simulink model "Relu_OutFB_4_4_1_HW_C1"  (R2012b)
settings: Solver=FixedStepDiscrete  SolverMode=SingleTasking  StartTime=0.0  StopTime=limSim*buffer  RelTol=1e-3
undefined symbols (not defined in the file): alpha, buffer, delayMulx, delayMuly, delayROMSig, limSim, m, M2, M3, magnitude, mu, n, p, ts
libraries: xbsIndex_r4 x268, dspstat3 x1, roblocks x1
(part 1 of 3)
settings Model: Creator=Marcelo  LastModifiedBy=snata
settings DataIOCC: SignalLoggingSaveFormat=ModelDataLogs
settings DebuggingCC: MultiTaskDSMMsg=warning  MultiTaskCondExecSysMsg=none  FcnCallInpInsideContextMsg=UseLocalSettings  StrictBusMsg=None
settings RTWCC: IncludeERTFirstTime=on
settings CodeAppCC: CustomSymbolStrType=$N$R$M_T  InternalIdentifier=Shortened
settings GRTTargetCC: CombineOutputUpdateFcns=off  GRTInterface=on

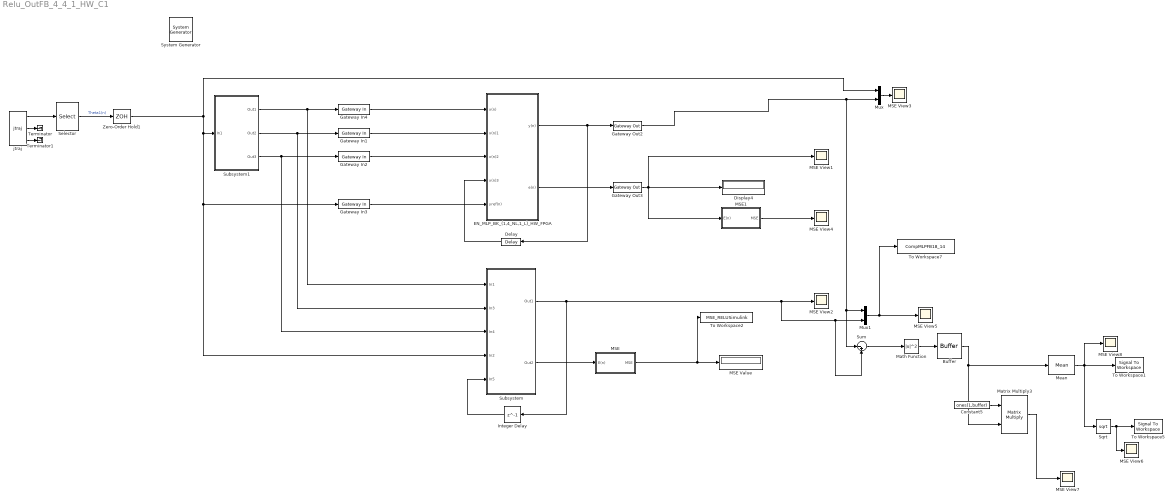
== system Relu_OutFB_4_4_1_HW_C1 ==
  " System Generator" : xbsIndex_r4/ System Generator  Tag=genX  xilinxfamily=virtex6  part=xc6vlx240t  speed=-1  package=ff1156  synthesis_tool=XST  clock_wrapper=Clock Enables  directory=C:/Users/snata/Documents/Netlist_MLP_Relu4_4_1  proj_type=Project Navigator  Synth_file=XST Defaults  Impl_file=ISE Defaults  testbench=off  simulink_period=ts  sysclk_period=10  dcm_input_clock_period=10  incr_netlist=off  trim_vbits=Everywhere in SubSystem  dbl_ovrd=According to Block Masks  core_generation=According to Block Masks  run_coregen=off  deprecated_control=off  eval_field=0  block_type=sysgen
  Buffer : Buffer  N=buffer  TreatMby1Signals=One channel
  Constant5 : Constant  Value=ones(1,buffer)  VectorParams1D=off
  Delay : xbsIndex_r4/Delay  rst=off  infoeditControl=Selection of Reset will increase slice count due to use of real FFs and instead of SRLs  en=off  latency=delayROMSig+delayMulx+delayMuly  dbl_ovrd=off  reg_retiming=off  block_type=delay
  Display4 : Display
  EN_MLP_BK_(1,4_NL,1_L)_HW_FPGA : Subsystem
  Gateway In{1..4} (4 alike) : xbsIndex_r4/Gateway In  gui_display_data_type=Fixed-point  arith_type="Signed  (2's comp)"  n_bits=nb  bin_pt=bp  preci_type=Single  exp_width=8  frac_width=24  quantization="Round  (unbiased: +/- Inf)"  overflow=Saturate  period=ts  dbl_ovrd=off  timing_constraint=None  locs_specified=off  LOCs={}  UseAsADC=off  ADCChannel='1'  inherit_from_input=off  hdl_port=on  block_type=gatewayin
  Gateway Out2 : xbsIndex_r4/Gateway Out  inherit_from_input=off  hdl_port=on  timing_constraint=None  locs_specified=off  LOCs={}  UseAsDAC=off  DACChannel='1'  block_type=gatewayout
      settings: infoedit="Gateway out block.  Converts Xilinx fixed point inputs into ouputs of type Simulink integer, double, or fixed point.<br><br>Hardware notes:  In hardware these blocks become top level output ports or are discarded, depending on how they are configured."
  Gateway Out3 : xbsIndex_r4/Gateway Out  inherit_from_input=off  hdl_port=on  timing_constraint=None  locs_specified=off  LOCs={}  UseAsDAC=off  DACChannel='1'  block_type=gatewayout
      settings: infoedit="Gateway out block.  Converts Xilinx fixed point inputs into ouputs of type Simulink integer, double, or fixed point.<br><br>Hardware notes:  In hardware these blocks become top level output ports or are discarded, depending on how they are configured."
  Integer Delay : Delay  DelayLength=1  InputProcessing=Inherited  SampleTime=ts
  MSE : Subsystem  mask(MSE){N=1, m=1}
      mask prompts: N "training size:"; m "Number of output neurons:"
      mask help:
      | MSE
      |
      | Prof. Marcelo Augusto Costa Fernandes
      | DCA - CT - UFRN
      | mfernandes@dca.ufrn.br
      mask Help:
      | MSE
      | 
      | Prof. Marcelo Augusto Costa Fernandes
      | DCA - CT - UFRN
      | mfernandes@dca.ufrn.br
  MSE Value : Display
  MSE View{1..8} (8 alike) : Scope
      MSE View1 settings: YMin=-70  YMax=70  SaveName=ScopeData2  MaxDataPoints=5000000
      MSE View2 settings: YMin=0.043  YMax=0.066  MaxDataPoints=5000000
      MSE View3 settings: ShowLegends=on  YMin=-70  YMax=70  SaveName=ScopeData7  MaxDataPoints=5000000
      MSE View4 settings: YMin=0.013  YMax=0.025  SaveName=ScopeData3  MaxDataPoints=5000000
      MSE View5 settings: YMin=-70  YMax=70  MaxDataPoints=5000000
      MSE View6 settings: TimeRange=1600  YMin=0.3388218390804599  YMax=0.5988218390804599  SaveName=ScopeData4  MaxDataPoints=5000000
      MSE View7 settings: TimeRange=1600  YMin=0.3388218390804599  YMax=0.5988218390804599  SaveName=ScopeData5  MaxDataPoints=5000000
      MSE View8 settings: TimeRange=1600  YMin=0.3388218390804599  YMax=0.5988218390804599  SaveName=ScopeData6  MaxDataPoints=5000000
  MSE1 : Subsystem  mask(MSE){N=1, m=1}
      mask prompts: N "training size:"; m "Number of output neurons:"
      mask help:
      | MSE
      |
      | Prof. Marcelo Augusto Costa Fernandes
      | DCA - CT - UFRN
      | mfernandes@dca.ufrn.br
      mask Help:
      | MSE
      | 
      | Prof. Marcelo Augusto Costa Fernandes
      | DCA - CT - UFRN
      | mfernandes@dca.ufrn.br
  Math Function : Math  Operator=magnitude^2  SaturateOnIntegerOverflow=on
  Matrix Multiply3 : Product  Multiplication=Matrix(*)
  Mean : dspstat3/Mean  run=off  reset_popup=None  InputProcessing=Columns as channels (frame based)  directionMode=Each column  dimension=1  treatSBRowAsCol=on  roiEnable=off  roiType=Rectangles  roiPortion=Entire ROI  roiOutput=Individual statistics for each ROI  roiFlag=off  outputDataTypeStr=Inherit: Same as accumulator  outputLastDataTypeStr=Inherit: Same as accumulator  outputMin=[]  outputMax=[]  roundingMode=Floor  overflowMode=off
  Mux : Mux  Inputs=2
  Mux1 : Mux  Inputs=2
  Selector : Selector  InputPortWidth=3  IndexOptions=Index vector (dialog)  Indices=[1]  OutputSizes=1
  Sqrt : Sqrt  SaturateOnIntegerOverflow=on
  Subsystem : Subsystem
  Subsystem1 : Subsystem
  Sum : Sum  Inputs=|-+
  Terminator : Terminator
  Terminator1 : Terminator
  To Workspace1 : SignalToWorkspace  VariableName=MSEMLPFB14_10
  To Workspace2 : ToWorkspace  VariableName=MSE_RELUSimulink  SampleTime=-1
  To Workspace5 : SignalToWorkspace  VariableName=RMSEMLPFB14_10
  To Workspace7 : ToWorkspace  VariableName=CompMLPFB18_14  SampleTime=-1
  Zero-Order Hold1 : ZeroOrderHold  SampleTime=ts
  jtraj : roblocks/Trajectory/jtraj  q0=[0 -pi/2 pi]  qf=[pi/2 pi/4 pi/2]  tmax=limSim*buffer  ts=1
  wires:
  jtraj/1 -> Selector/1
  Selector/1 -> Zero-Order Hold1/1  "Theta1(n)"
  jtraj/2 -> Terminator/1
  jtraj/3 -> Terminator1/1
  EN_MLP_BK_(1,4_NL,1_L)_HW_FPGA/2(e(n)) -> Gateway Out3/1
  Gateway In4/1 -> EN_MLP_BK_(1,4_NL,1_L)_HW_FPGA/1(x(n))
  Gateway In3/1 -> EN_MLP_BK_(1,4_NL,1_L)_HW_FPGA/5(yref(n))
  Gateway Out3/1 -> MSE1/1(E(n)), MSE View1/1, Display4/1
  Gateway In1/1 -> EN_MLP_BK_(1,4_NL,1_L)_HW_FPGA/2(x(n)1)
  Gateway In2/1 -> EN_MLP_BK_(1,4_NL,1_L)_HW_FPGA/3(x(n)2)
  MSE1/1(MSE) -> MSE View4/1
  EN_MLP_BK_(1,4_NL,1_L)_HW_FPGA/1(y(n)) -> Delay/1, Gateway Out2/1
  Delay/1 -> EN_MLP_BK_(1,4_NL,1_L)_HW_FPGA/4(x(n)3)
  Mux/1 -> MSE View3/1
  Subsystem1/1(Out1) -> Subsystem/1(In1), Gateway In4/1
  Subsystem1/2(Out2) -> Subsystem/2(In3), Gateway In1/1
  Subsystem1/3(Out3) -> Subsystem/3(In4), Gateway In2/1
  Subsystem/2(Out2) -> MSE/1(E(n))
  Zero-Order Hold1/1 -> Subsystem1/1(In1), Subsystem/4(In2), Gateway In3/1, Mux/1
  Mux1/1 -> MSE View5/1, To Workspace7/1
  MSE/1(MSE) -> To Workspace2/1, MSE Value/1
  Integer Delay/1 -> Subsystem/5(In5)
  Sum/1 -> Math Function/1
  Math Function/1 -> Buffer/1
  Buffer/1 -> Mean/1, Matrix Multiply3/2
  Mean/1 -> MSE View8/1, Sqrt/1, To Workspace1/1
  Matrix Multiply3/1 -> MSE View7/1
  Constant5/1 -> Matrix Multiply3/1
  Sqrt/1 -> MSE View6/1, To Workspace5/1
  Gateway Out2/1 -> Sum/1, Mux1/1, Mux/2
  Subsystem/1(Out1) -> Integer Delay/1, Sum/2, Mux1/2, MSE View2/1

== system Relu_OutFB_4_4_1_HW_C1/EN_MLP_BK_(1,4_NL,1_L)_HW_FPGA ==
  x(n) : Inport
  x(n)1 : Inport  Port=2
  x(n)2 : Inport  Port=3
  x(n)3 : Inport  Port=4
  yref(n) : Inport  Port=5
  MLP_BK_(2,4_NL,1_L)_HW_FPGA : Subsystem
  y(n) : Outport
  e(n) : Outport  Port=2
  wires:
  yref(n)/1 -> MLP_BK_(2,4_NL,1_L)_HW_FPGA/5(y_ref(n))
  x(n)/1 -> MLP_BK_(2,4_NL,1_L)_HW_FPGA/1(x_1(n))  "x(n)"
  MLP_BK_(2,4_NL,1_L)_HW_FPGA/2(e(n)) -> e(n)/1
  x(n)1/1 -> MLP_BK_(2,4_NL,1_L)_HW_FPGA/2(x_2(n))
  x(n)2/1 -> MLP_BK_(2,4_NL,1_L)_HW_FPGA/3(x_3(n))
  MLP_BK_(2,4_NL,1_L)_HW_FPGA/1(y(n)) -> y(n)/1
  x(n)3/1 -> MLP_BK_(2,4_NL,1_L)_HW_FPGA/4(x_4(n))

== system Relu_OutFB_4_4_1_HW_C1/MSE ==
  E(n) : Inport
  Add1 : Sum  Inputs=1
  Constant5 : Constant  Value=ones(1,m)  VectorParams1D=off
  Gain : Gain  Gain=1/N
  Math Function : Math  Operator=magnitude^2  SaturateOnIntegerOverflow=on
  Matrix Multiply3 : Product  Multiplication=Matrix(*)
  MSE : Outport
  wires:
  Add1/1 -> Gain/1
  Constant5/1 -> Matrix Multiply3/1
  Math Function/1 -> Matrix Multiply3/2
  Matrix Multiply3/1 -> Add1/1
  E(n)/1 -> Math Function/1
  Gain/1 -> MSE/1

== system Relu_OutFB_4_4_1_HW_C1/MSE1 ==
  E(n) : Inport
  Add1 : Sum  Inputs=1
  Constant5 : Constant  Value=ones(1,m)  VectorParams1D=off
  Gain : Gain  Gain=1/N
  Math Function : Math  Operator=magnitude^2  SaturateOnIntegerOverflow=on
  Matrix Multiply3 : Product  Multiplication=Matrix(*)
  MSE : Outport
  wires:
  Gain/1 -> MSE/1
  E(n)/1 -> Math Function/1
  Matrix Multiply3/1 -> Add1/1
  Math Function/1 -> Matrix Multiply3/2
  Constant5/1 -> Matrix Multiply3/1
  Add1/1 -> Gain/1

== system Relu_OutFB_4_4_1_HW_C1/Subsystem ==
  In1 : Inport
  In3 : Inport  Port=2
  In4 : Inport  Port=3
  In2 : Inport  Port=4
  In5 : Inport  Port=5
  Add : Sum  Inputs=-+|
  Backpropagation Algorithm : Subsystem  mask(Backpropagation Algorithm){mu=mu, alpha=0, N=1, p=n, H=m, m=p, ts=ts}
      mask prompts: N "training size:"; p "Number of the inputs:"; H "Number of hidden neurons:"; m "Number of output neurons:"; ts "Sample time:"
      mask help:
      | Backpropagation Algorithm
      |
      | Prof. Marcelo A. C. Fernandes
      | DCA - CT - UFRN
      | mfernandes@dca.ufrn.br
      mask Help:
      | Backpropagation Algorithm
      | 
      | Prof. Marcelo A. C. Fernandes
      | DCA - CT - UFRN
      | mfernandes@dca.ufrn.br
  MLP - 2 Layers : Subsystem  mask(Multilayer Perceptron (MLP) - 2 Layers){N=1, valorLimiar=1, p=n, H=m, m=p, ts=ts}
      mask prompts: N "training size:"; valorLimiar "Bias value:"; p "Number of the inputs:"; H "Number of hidden neurons:"; m "Number of output neurons:"; ts "sampleTime"
      mask help:
      | Multilayer Perceptron (MLP) - 2 Layers
      |
      | Prof. Marcelo Augusto Costa Fernandes
      | DCA - CT - UFRN
      | mfernandes@dca.ufrn.br
      mask Help:
      | Multilayer Perceptron (MLP) - 2 Layers
      | 
      | Prof. Marcelo Augusto Costa Fernandes
      | DCA - CT - UFRN
      | mfernandes@dca.ufrn.br
  Matrix Concatenate : Concatenate  NumInputs=4  Mode=Multidimensional array
  Out1 : Outport
  Out2 : Outport  Port=2
  wires:
  MLP - 2 Layers/1(Y(n)) -> Add/1, Out1/1
  In4/1 -> Matrix Concatenate/3
  In3/1 -> Matrix Concatenate/2
  In1/1 -> Matrix Concatenate/1
  In2/1 -> Add/2
  Matrix Concatenate/1 -> MLP - 2 Layers/1(X(n))
  Backpropagation Algorithm/1(Wy(n+1)) -> MLP - 2 Layers/3(Wy(n+1))
  Add/1 -> Out2/1, Backpropagation Algorithm/3(E(n))
  MLP - 2 Layers/2("[bias|Z(n)]") -> Backpropagation Algorithm/2("[bias|Z(n)]")
  MLP - 2 Layers/3("[bias|X(n)]") -> Backpropagation Algorithm/1("[bias|X(n)]")
  In5/1 -> Matrix Concatenate/4
  Backpropagation Algorithm/2(Wx(n+1)) -> MLP - 2 Layers/2(Wx(n+1))

== system Relu_OutFB_4_4_1_HW_C1/Subsystem1 ==
  In1 : Inport
  Delay{1..6} (6 alike) : Delay  DelayLength=1
  Terminator : Terminator
  Out1 : Outport
  Out2 : Outport  Port=2
  Out3 : Outport  Port=3
  wires:
  Delay4/1 -> Delay1/1, Out3/1
  Delay2/1 -> Out2/1, Delay4/1
  Delay3/1 -> Out1/1, Delay2/1
  In1/1 -> Delay3/1
  Delay1/1 -> Delay5/1
  Delay5/1 -> Delay6/1
  Delay6/1 -> Terminator/1

== system Relu_OutFB_4_4_1_HW_C1/EN_MLP_BK_(1,4_NL,1_L)_HW_FPGA/MLP_BK_(2,4_NL,1_L)_HW_FPGA ==
  x_1(n) : Inport
  x_2(n) : Inport  Port=2
  x_3(n) : Inport  Port=3
  x_4(n) : Inport  Port=4
  y_ref(n) : Inport  Port=5
  AddSub : xbsIndex_r4/AddSub  mode=Subtraction  use_carryin=off  use_carryout=off  en=off  latency=0  precision=User Defined  arith_type="Signed  (2's comp)"  n_bits=nb  bin_pt=bp  quantization="Round  (unbiased: +/- Inf)"  overflow=Wrap  dbl_ovrd=off  use_behavioral_HDL=off  hw_selection=Fabric  pipelined=off  block_type=addsub
  BK (2,4_NL,1_L) : Subsystem
  Delay{,1..4} (5 alike) : xbsIndex_r4/Delay  rst=off  infoeditControl=Selection of Reset will increase slice count due to use of real FFs and instead of SRLs  en=off  latency=delayROMSig+delayMulx+delayMuly  dbl_ovrd=off  reg_retiming=off  block_type=delay
  MLP (2,4_NL,1_L) : Subsystem
  y(n) : Outport
  e(n) : Outport  Port=2
  wires:
  Delay/1 -> AddSub/1
  y_ref(n)/1 -> Delay/1
  x_1(n)/1 -> MLP (2,4_NL,1_L)/4(x_1(n))
  BK (2,4_NL,1_L)/1(Wy_10(n)) -> MLP (2,4_NL,1_L)/29(Wy_10(n))
  AddSub/1 -> e(n)/1, BK (2,4_NL,1_L)/11(e(n))
  BK (2,4_NL,1_L)/2(Wy_11(n)) -> MLP (2,4_NL,1_L)/28(Wy_11(n))
  x_2(n)/1 -> MLP (2,4_NL,1_L)/3(x_2(n))
  x_3(n)/1 -> MLP (2,4_NL,1_L)/2(x_3(n))
  x_4(n)/1 -> MLP (2,4_NL,1_L)/1(x_4(n))
  BK (2,4_NL,1_L)/3(Wy_12(n)) -> MLP (2,4_NL,1_L)/27(Wy_12(n))
  BK (2,4_NL,1_L)/4(Wy_13(n)) -> MLP (2,4_NL,1_L)/26(Wy_13(n))
  BK (2,4_NL,1_L)/5(Wy_14(n)) -> MLP (2,4_NL,1_L)/25(Wy_14(n))
  BK (2,4_NL,1_L)/6(Wx_10(n)) -> MLP (2,4_NL,1_L)/24(Wx_10(n))
  BK (2,4_NL,1_L)/7(Wx_11(n)) -> MLP (2,4_NL,1_L)/23(Wx_11(n))
  BK (2,4_NL,1_L)/8(Wx_12(n)) -> MLP (2,4_NL,1_L)/22(Wx_12(n))
  BK (2,4_NL,1_L)/9(Wx_13(n)) -> MLP (2,4_NL,1_L)/21(Wx_13(n))
  BK (2,4_NL,1_L)/10(Wx_14(n)) -> MLP (2,4_NL,1_L)/20(Wx_14(n))
  BK (2,4_NL,1_L)/11(Wx_20(n)) -> MLP (2,4_NL,1_L)/19(Wx_20(n))
  BK (2,4_NL,1_L)/12(Wx_21(n)) -> MLP (2,4_NL,1_L)/18(Wx_21(n))
  BK (2,4_NL,1_L)/13(Wx_22(n)) -> MLP (2,4_NL,1_L)/17(Wx_22(n))
  BK (2,4_NL,1_L)/14(Wx_23(n)) -> MLP (2,4_NL,1_L)/16(Wx_23(n))
  BK (2,4_NL,1_L)/15(Wx_24(n)) -> MLP (2,4_NL,1_L)/15(Wx_24(n))
  BK (2,4_NL,1_L)/16(Wx_30(n)) -> MLP (2,4_NL,1_L)/14(Wx_30(n))
  BK (2,4_NL,1_L)/17(Wx_31(n)) -> MLP (2,4_NL,1_L)/13(Wx_31(n))
  BK (2,4_NL,1_L)/18(Wx_32(n)) -> MLP (2,4_NL,1_L)/12(Wx_32(n)1)
  BK (2,4_NL,1_L)/19(Wx_33(n)) -> MLP (2,4_NL,1_L)/11(Wx_33(n))
  BK (2,4_NL,1_L)/20(Wx_34(n)) -> MLP (2,4_NL,1_L)/10(Wx_34(n))
  BK (2,4_NL,1_L)/21(Wx_40(n)) -> MLP (2,4_NL,1_L)/9(Wx_40(n))
  BK (2,4_NL,1_L)/22(Wx_41(n)) -> MLP (2,4_NL,1_L)/8(Wx_41(n))
  BK (2,4_NL,1_L)/23(Wx_42(n)) -> MLP (2,4_NL,1_L)/7(Wx_42(n))
  BK (2,4_NL,1_L)/24(Wx_43(n)) -> MLP (2,4_NL,1_L)/6(Wx_43(n))
  BK (2,4_NL,1_L)/25(Wx_44(n)) -> MLP (2,4_NL,1_L)/5(Wx_44(n))
  MLP (2,4_NL,1_L)/11(x_4(n)bp) -> Delay1/1
  MLP (2,4_NL,1_L)/10(x_3(n)bp) -> Delay2/1
  MLP (2,4_NL,1_L)/9(x_2(n)bp) -> Delay3/1
  MLP (2,4_NL,1_L)/8(x_1(n)bp) -> Delay4/1
  MLP (2,4_NL,1_L)/6(z_4(n)) -> BK (2,4_NL,1_L)/6(z_4(n))
  MLP (2,4_NL,1_L)/5(z_3(n)) -> BK (2,4_NL,1_L)/7(z_3(n))
  MLP (2,4_NL,1_L)/4(z_2(n)) -> BK (2,4_NL,1_L)/8(z_2(n))
  MLP (2,4_NL,1_L)/3(z_1(n)) -> BK (2,4_NL,1_L)/9(z_1(n))
  MLP (2,4_NL,1_L)/2(z_0(n)) -> BK (2,4_NL,1_L)/10(z_0(n))
  MLP (2,4_NL,1_L)/1(y_0(n)) -> y(n)/1, AddSub/2
  Delay1/1 -> BK (2,4_NL,1_L)/1(x_4(n))
  Delay2/1 -> BK (2,4_NL,1_L)/2(x_3(n))
  Delay3/1 -> BK (2,4_NL,1_L)/3(x_2(n))
  Delay4/1 -> BK (2,4_NL,1_L)/4(x_1(n))
  MLP (2,4_NL,1_L)/7(x_0(n)bp) -> BK (2,4_NL,1_L)/5(x_0(n))

== system Relu_OutFB_4_4_1_HW_C1/Subsystem/Backpropagation Algorithm ==
  "[bias|X(n)]" : Inport
  "[bias|Z(n)]" : Inport  Port=2
  E(n) : Inport  Port=3
  Hidden Layer : Subsystem
  Output Layer : Subsystem
  Wy(n+1) : Outport
  Wx(n+1) : Outport  Port=2
  wires:
  Output Layer/1(Wy(n+1)) -> Wy(n+1)/1  "Wy(n+1)"
  "[bias|Z(n)]"/1 -> Output Layer/1("[bias|Z(n)]"), Hidden Layer/4("[bias|Z(n)]")  "[bias|Z(n)]"
  E(n)/1 -> Output Layer/2(E(n))  "E(n)"
  Output Layer/2(Wy(n)) -> Hidden Layer/1(Wy(n))  "Wy(n)"
  Output Layer/3(Gy(n)) -> Hidden Layer/2(Gy(n))  "Gy(n)"
  "[bias|X(n)]"/1 -> Hidden Layer/3("[bias|X(n)]")  "[bias|X(n)]"
  Hidden Layer/1(Wx(n+1)) -> Wx(n+1)/1

== system Relu_OutFB_4_4_1_HW_C1/Subsystem/MLP - 2 Layers ==
  X(n) : Inport
  Wx(n+1) : Inport  Port=2
  Wy(n+1) : Inport  Port=3
  Constant : Constant  Value=valorLimiar*ones(1,N)  VectorParams1D=off  SampleTime=ts
  Matrix Concatenation : Concatenate  Mode=Multidimensional array
  Matrix Concatenation1 : Concatenate  Mode=Multidimensional array
  Matrix Multiply : Product  Multiplication=Matrix(*)
  Matrix Multiply1 : Product  Multiplication=Matrix(*)
  Sigmoid : Subsystem  mask(Sigmoid Function){}
      mask help:
      | Sigmoid Function.
      |
      | 1/(1+exp(-x))
      |
      | Prof. Marcelo Fernandes
      | DCA - CT - UFRN
      | mfernandes@dca.ufrn.br
      mask Help:
      | Sigmoid Function.
      | 
      | 1/(1+exp(-x))
      | 
      | Prof. Marcelo Fernandes
      | DCA - CT - UFRN
      | mfernandes@dca.ufrn.br
      mask Display: plot([-8:.1:8],(1-exp(-1*[-8:.1:8]))./(1+exp(-1*[-8:.1:8])))
  Y(n) : Outport
  "[bias|Z(n)]" : Outport  Port=2
  "[bias|X(n)]" : Outport  Port=3
  wires:
  Constant/1 -> Matrix Concatenation/1, Matrix Concatenation1/1
  Matrix Concatenation/1 -> Matrix Multiply/2, "[bias|X(n)]"/1  "X"
  Matrix Multiply/1 -> Sigmoid/1(In1)  "V(n)"
  X(n)/1 -> Matrix Concatenation/2
  Wx(n+1)/1 -> Matrix Multiply/1
  Matrix Multiply1/1 -> Y(n)/1  "B(n)"
  Sigmoid/1(Out1) -> Matrix Concatenation1/2  "Z(n)"
  Matrix Concatenation1/1 -> Matrix Multiply1/2, "[bias|Z(n)]"/1
  Wy(n+1)/1 -> Matrix Multiply1/1

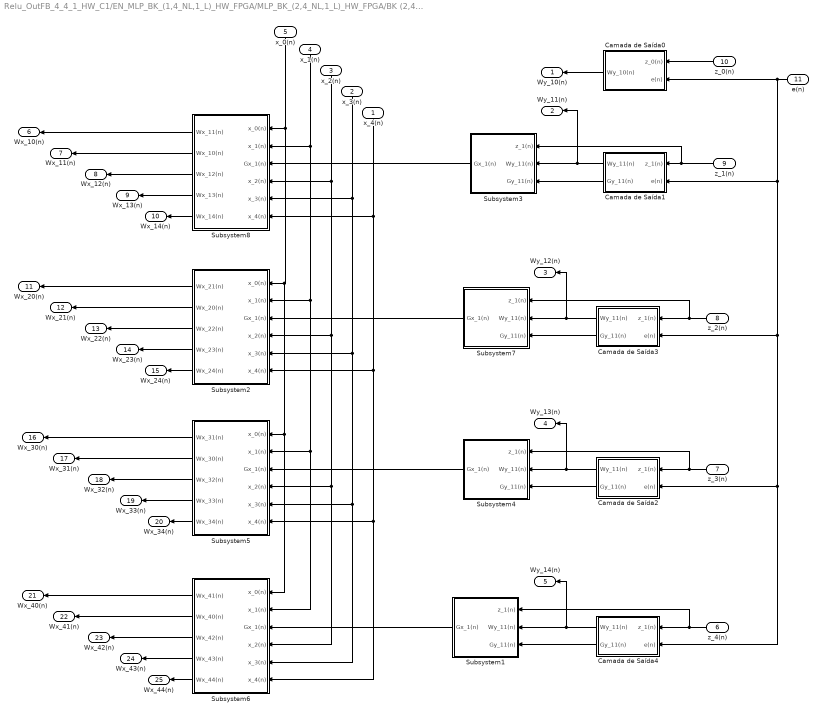
== system Relu_OutFB_4_4_1_HW_C1/EN_MLP_BK_(1,4_NL,1_L)_HW_FPGA/MLP_BK_(2,4_NL,1_L)_HW_FPGA/BK (2,4_NL,1_L) ==
  x_4(n) : Inport
  x_3(n) : Inport  Port=2
  x_2(n) : Inport  Port=3
  x_1(n) : Inport  Port=4
  x_0(n) : Inport  Port=5
  z_4(n) : Inport  Port=6
  z_3(n) : Inport  Port=7
  z_2(n) : Inport  Port=8
  z_1(n) : Inport  Port=9
  z_0(n) : Inport  Port=10
  e(n) : Inport  Port=11
  Camada de Saída0 : Subsystem
  Camada de Saída1 : Subsystem
  Camada de Saída2 : Subsystem
  Camada de Saída3 : Subsystem
  Camada de Saída4 : Subsystem
  Subsystem1 : Subsystem
  Subsystem2 : Subsystem
  Subsystem3 : Subsystem
  Subsystem4 : Subsystem
  Subsystem5 : Subsystem
  Subsystem6 : Subsystem
  Subsystem7 : Subsystem
  Subsystem8 : Subsystem
  Wy_10(n) : Outport
  Wy_11(n) : Outport  Port=2
  Wy_12(n) : Outport  Port=3
  Wy_13(n) : Outport  Port=4
  Wy_14(n) : Outport  Port=5
  Wx_10(n) : Outport  Port=6
  Wx_11(n) : Outport  Port=7
  Wx_12(n) : Outport  Port=8
  Wx_13(n) : Outport  Port=9
  Wx_14(n) : Outport  Port=10
  Wx_20(n) : Outport  Port=11
  Wx_21(n) : Outport  Port=12
  Wx_22(n) : Outport  Port=13
  Wx_23(n) : Outport  Port=14
  Wx_24(n) : Outport  Port=15
  Wx_30(n) : Outport  Port=16
  Wx_31(n) : Outport  Port=17
  Wx_32(n) : Outport  Port=18
  Wx_33(n) : Outport  Port=19
  Wx_34(n) : Outport  Port=20
  Wx_40(n) : Outport  Port=21
  Wx_41(n) : Outport  Port=22
  Wx_42(n) : Outport  Port=23
  Wx_43(n) : Outport  Port=24
  Wx_44(n) : Outport  Port=25
  wires:
  e(n)/1 -> Camada de Saída0/2(e(n)), Camada de Saída1/2(e(n)), Camada de Saída4/2(e(n)), Camada de Saída2/2(e(n)), Camada de Saída3/2(e(n))
  Camada de Saída0/1(Wy_10(n)) -> Wy_10(n)/1
  z_1(n)/1 -> Subsystem3/1(z_1(n)), Camada de Saída1/1(z_1(n))
  z_0(n)/1 -> Camada de Saída0/1(z_0(n))
  Camada de Saída1/1(Wy_11(n)) -> Wy_11(n)/1, Subsystem3/2(Wy_11(n))
  Subsystem3/1(Gx_1(n)) -> Subsystem8/3(Gx_1(n))
  Subsystem8/1(Wx_11(n)) -> Wx_10(n)/1
  Subsystem8/2(Wx_10(n)) -> Wx_11(n)/1
  z_2(n)/1 -> Subsystem7/1(z_1(n)), Camada de Saída3/1(z_1(n))
  Camada de Saída3/2(Gy_11(n)) -> Subsystem7/3(Gy_11(n))
  Camada de Saída3/1(Wy_11(n)) -> Subsystem7/2(Wy_11(n)), Wy_12(n)/1
  z_3(n)/1 -> Subsystem4/1(z_1(n)), Camada de Saída2/1(z_1(n))
  Camada de Saída2/2(Gy_11(n)) -> Subsystem4/3(Gy_11(n))
  Camada de Saída2/1(Wy_11(n)) -> Subsystem4/2(Wy_11(n)), Wy_13(n)/1
  z_4(n)/1 -> Subsystem1/1(z_1(n)), Camada de Saída4/1(z_1(n))
  Camada de Saída4/2(Gy_11(n)) -> Subsystem1/3(Gy_11(n))
  Camada de Saída4/1(Wy_11(n)) -> Subsystem1/2(Wy_11(n)), Wy_14(n)/1
  Subsystem1/1(Gx_1(n)) -> Subsystem6/3(Gx_1(n))
  Subsystem8/3(Wx_12(n)) -> Wx_12(n)/1
  Subsystem8/4(Wx_13(n)) -> Wx_13(n)/1
  Subsystem8/5(Wx_14(n)) -> Wx_14(n)/1
  Subsystem7/1(Gx_1(n)) -> Subsystem2/3(Gx_1(n))
  x_1(n)/1 -> Subsystem8/2(x_1(n)), Subsystem2/2(x_1(n)), Subsystem6/2(x_1(n)), Subsystem5/2(x_1(n))
  x_0(n)/1 -> Subsystem8/1(x_0(n)), Subsystem2/1(x_0(n)), Subsystem6/1(x_0(n)), Subsystem5/1(x_0(n))
  x_3(n)/1 -> Subsystem8/5(x_3(n)), Subsystem2/5(x_3(n)), Subsystem5/5(x_3(n)), Subsystem6/5(x_3(n))
  x_2(n)/1 -> Subsystem8/4(x_2(n)), Subsystem2/4(x_2(n)), Subsystem5/4(x_2(n)), Subsystem6/4(x_2(n))
  x_4(n)/1 -> Subsystem8/6(x_4(n)), Subsystem2/6(x_4(n)), Subsystem5/6(x_4(n)), Subsystem6/6(x_4(n))
  Subsystem4/1(Gx_1(n)) -> Subsystem5/3(Gx_1(n))
  Subsystem2/1(Wx_21(n)) -> Wx_20(n)/1
  Subsystem2/2(Wx_20(n)) -> Wx_21(n)/1
  Subsystem2/3(Wx_22(n)) -> Wx_22(n)/1
  Subsystem2/4(Wx_23(n)) -> Wx_23(n)/1
  Subsystem2/5(Wx_24(n)) -> Wx_24(n)/1
  Subsystem5/1(Wx_31(n)) -> Wx_30(n)/1
  Subsystem5/2(Wx_30(n)) -> Wx_31(n)/1
  Subsystem5/3(Wx_32(n)) -> Wx_32(n)/1
  Subsystem5/4(Wx_33(n)) -> Wx_33(n)/1
  Subsystem5/5(Wx_34(n)) -> Wx_34(n)/1
  Subsystem6/1(Wx_41(n)) -> Wx_40(n)/1
  Subsystem6/2(Wx_40(n)) -> Wx_41(n)/1
  Subsystem6/3(Wx_42(n)) -> Wx_42(n)/1
  Subsystem6/4(Wx_43(n)) -> Wx_43(n)/1
  Subsystem6/5(Wx_44(n)) -> Wx_44(n)/1
  Camada de Saída1/2(Gy_11(n)) -> Subsystem3/3(Gy_11(n))

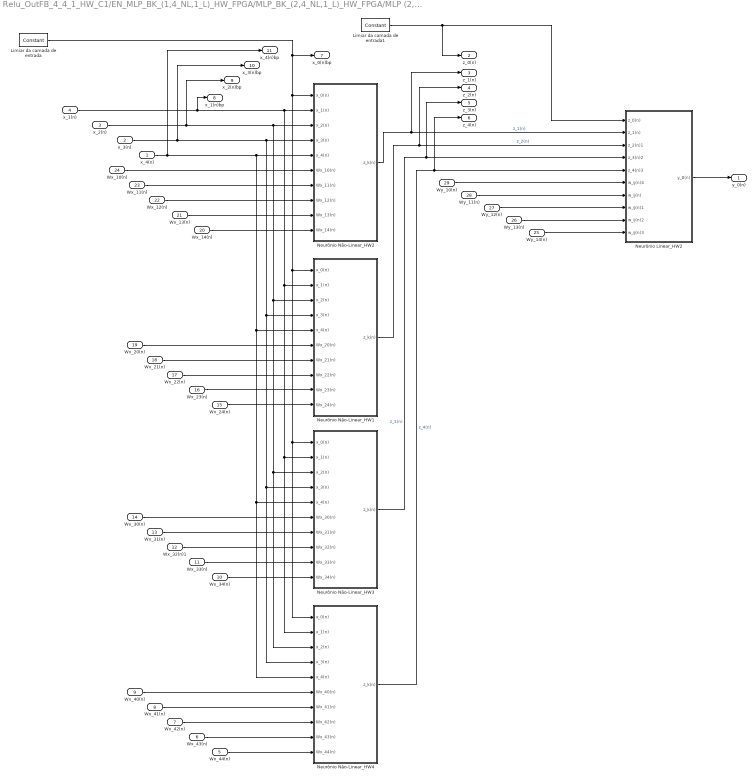
== system Relu_OutFB_4_4_1_HW_C1/EN_MLP_BK_(1,4_NL,1_L)_HW_FPGA/MLP_BK_(2,4_NL,1_L)_HW_FPGA/MLP (2,4_NL,1_L) ==
  x_4(n) : Inport
  x_3(n) : Inport  Port=2
  x_2(n) : Inport  Port=3
  x_1(n) : Inport  Port=4
  Wx_44(n) : Inport  Port=5
  Wx_43(n) : Inport  Port=6
  Wx_42(n) : Inport  Port=7
  Wx_41(n) : Inport  Port=8
  Wx_40(n) : Inport  Port=9
  Wx_34(n) : Inport  Port=10
  Wx_33(n) : Inport  Port=11
  Wx_32(n)1 : Inport  Port=12
  Wx_31(n) : Inport  Port=13
  Wx_30(n) : Inport  Port=14
  Wx_24(n) : Inport  Port=15
  Wx_23(n) : Inport  Port=16
  Wx_22(n) : Inport  Port=17
  Wx_21(n) : Inport  Port=18
  Wx_20(n) : Inport  Port=19
  Wx_14(n) : Inport  Port=20
  Wx_13(n) : Inport  Port=21
  Wx_12(n) : Inport  Port=22
  Wx_11(n) : Inport  Port=23
  Wx_10(n) : Inport  Port=24
  Wy_14(n) : Inport  Port=25
  Wy_13(n) : Inport  Port=26
  Wy_12(n) : Inport  Port=27
  Wy_11(n) : Inport  Port=28
  Wy_10(n) : Inport  Port=29
  Limiar da camada de entrada : xbsIndex_r4/Constant  const=1  gui_display_data_type=Fixed-point  arith_type=Signed (2's comp)  n_bits=nb  bin_pt=bp  preci_type=Single  exp_width=8  frac_width=24  explicit_period=off  period=0.01  equ=P=C  opselect=C  inp2=PCIN>>17  opr=+  inp1=P  carry=CIN  dbl_ovrd=off  block_type=constant
  Limiar da camada de entrada1 : xbsIndex_r4/Constant  const=1  gui_display_data_type=Fixed-point  arith_type=Signed (2's comp)  n_bits=nb  bin_pt=bp  preci_type=Single  exp_width=8  frac_width=24  explicit_period=off  period=0.01  equ=P=C  opselect=C  inp2=PCIN>>17  opr=+  inp1=P  carry=CIN  dbl_ovrd=off  block_type=constant
  Neurônio Linear_HW2 : Subsystem
  Neurônio Não-Linear_HW1 : Subsystem
  Neurônio Não-Linear_HW2 : Subsystem
  Neurônio Não-Linear_HW3 : Subsystem
  Neurônio Não-Linear_HW4 : Subsystem
  y_0(n) : Outport
  z_0(n) : Outport  Port=2
  z_1(n) : Outport  Port=3
  z_2(n) : Outport  Port=4
  z_3(n) : Outport  Port=5
  z_4(n) : Outport  Port=6
  x_0(n)bp : Outport  Port=7
  x_1(n)bp : Outport  Port=8
  x_2(n)bp : Outport  Port=9
  x_3(n)bp : Outport  Port=10
  x_4(n)bp : Outport  Port=11
  wires:
  Wy_14(n)/1 -> Neurônio Linear_HW2/10(w_ij(n)3)
  Wy_13(n)/1 -> Neurônio Linear_HW2/9(w_ij(n)2)
  Wy_12(n)/1 -> Neurônio Linear_HW2/8(w_ij(n)1)
  Wy_11(n)/1 -> Neurônio Linear_HW2/7(w_ij(n))
  Wy_10(n)/1 -> Neurônio Linear_HW2/6(w_ij(n)4)
  Wx_41(n)/1 -> Neurônio Não-Linear_HW4/7(Wx_41(n))
  Wx_40(n)/1 -> Neurônio Não-Linear_HW4/6(Wx_40(n))
  Limiar da camada de entrada/1 -> Neurônio Não-Linear_HW2/1(x_0(n)), Neurônio Não-Linear_HW4/1(x_0(n)), Neurônio Não-Linear_HW3/1(x_0(n)), Neurônio Não-Linear_HW1/1(x_0(n)), x_0(n)bp/1
  Neurônio Não-Linear_HW4/1(z_k(n)) -> Neurônio Linear_HW2/5(z_4(n)3), z_4(n)/1  "z_4(n)"
  Neurônio Não-Linear_HW3/1(z_k(n)) -> Neurônio Linear_HW2/4(z_3(n)2), z_3(n)/1  "z_3(n)"
  Neurônio Não-Linear_HW2/1(z_k(n)) -> Neurônio Linear_HW2/2(z_1(n)), z_1(n)/1  "z_1(n)"
  Neurônio Linear_HW2/1(y_0(n)) -> y_0(n)/1
  Neurônio Não-Linear_HW1/1(z_k(n)) -> Neurônio Linear_HW2/3(z_2(n)1), z_2(n)/1  "z_2(n)"
  Wx_43(n)/1 -> Neurônio Não-Linear_HW4/9(Wx_43(n))
  Wx_42(n)/1 -> Neurônio Não-Linear_HW4/8(Wx_42(n))
  Wx_44(n)/1 -> Neurônio Não-Linear_HW4/10(Wx_44(n))
  Wx_31(n)/1 -> Neurônio Não-Linear_HW3/7(Wx_31(n))
  Wx_30(n)/1 -> Neurônio Não-Linear_HW3/6(Wx_30(n))
  Wx_33(n)/1 -> Neurônio Não-Linear_HW3/9(Wx_33(n))
  Wx_32(n)1/1 -> Neurônio Não-Linear_HW3/8(Wx_32(n))
  Wx_34(n)/1 -> Neurônio Não-Linear_HW3/10(Wx_34(n))
  Wx_21(n)/1 -> Neurônio Não-Linear_HW1/7(Wx_21(n))
  Wx_20(n)/1 -> Neurônio Não-Linear_HW1/6(Wx_20(n))
  Wx_23(n)/1 -> Neurônio Não-Linear_HW1/9(Wx_23(n))
  Wx_22(n)/1 -> Neurônio Não-Linear_HW1/8(Wx_22(n))
  Wx_24(n)/1 -> Neurônio Não-Linear_HW1/10(Wx_24(n))
  Wx_11(n)/1 -> Neurônio Não-Linear_HW2/7(Wx_11(n))
  Wx_10(n)/1 -> Neurônio Não-Linear_HW2/6(Wx_10(n))
  Wx_13(n)/1 -> Neurônio Não-Linear_HW2/9(Wx_13(n))
  Wx_12(n)/1 -> Neurônio Não-Linear_HW2/8(Wx_12(n))
  Wx_14(n)/1 -> Neurônio Não-Linear_HW2/10(Wx_14(n))
  x_1(n)/1 -> Neurônio Não-Linear_HW2/2(x_1(n)), Neurônio Não-Linear_HW4/2(x_1(n)), Neurônio Não-Linear_HW3/2(x_1(n)), Neurônio Não-Linear_HW1/2(x_1(n)), x_1(n)bp/1
  x_2(n)/1 -> Neurônio Não-Linear_HW4/3(x_2(n)), Neurônio Não-Linear_HW3/3(x_2(n)), Neurônio Não-Linear_HW1/3(x_2(n)), Neurônio Não-Linear_HW2/3(x_2(n)), x_2(n)bp/1
  x_3(n)/1 -> x_3(n)bp/1, Neurônio Não-Linear_HW4/4(x_3(n)), Neurônio Não-Linear_HW3/4(x_3(n)), Neurônio Não-Linear_HW1/4(x_3(n)), Neurônio Não-Linear_HW2/4(x_3(n))
  x_4(n)/1 -> x_4(n)bp/1, Neurônio Não-Linear_HW4/5(x_4(n)), Neurônio Não-Linear_HW3/5(x_4(n)), Neurônio Não-Linear_HW1/5(x_4(n)), Neurônio Não-Linear_HW2/5(x_4(n))
  Limiar da camada de entrada1/1 -> Neurônio Linear_HW2/1(z_0(n)), z_0(n)/1

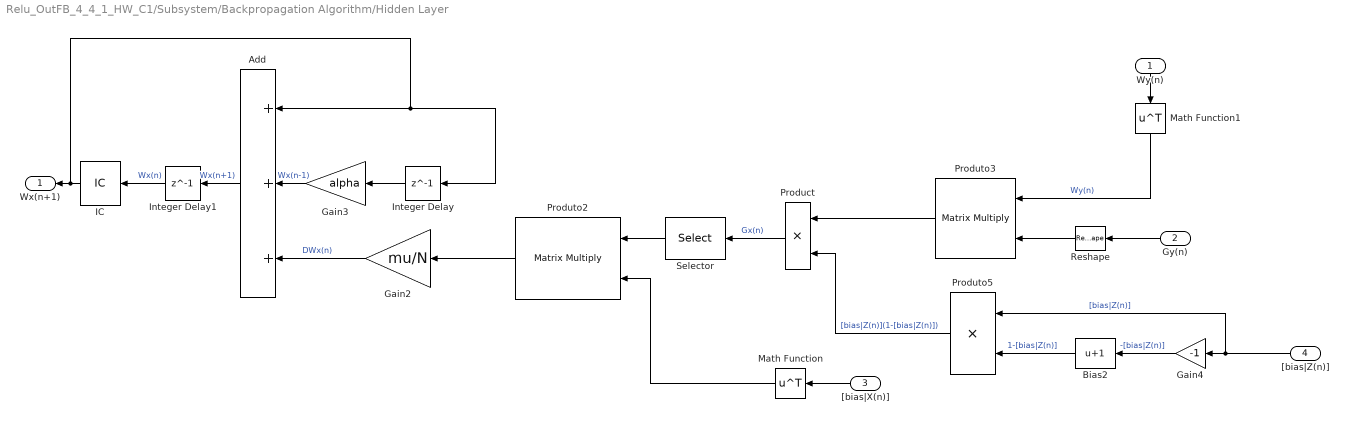
== system Relu_OutFB_4_4_1_HW_C1/Subsystem/Backpropagation Algorithm/Hidden Layer ==
  Wy(n) : Inport
  Gy(n) : Inport  Port=2
  "[bias|X(n)]" : Inport  Port=3
  "[bias|Z(n)]" : Inport  Port=4
  Add : Sum  Inputs=+++
  Bias2 : Bias  Bias=1
  Gain2 : Gain  Gain=mu/N
  Gain3 : Gain  Gain=alpha
  Gain4 : Gain  Gain=-1
  IC : InitialCondition  Value=rand(H,p+1)
  Integer Delay : Delay  DelayLength=1  InputProcessing=Inherited  SampleTime=ts
  Integer Delay1 : Delay  DelayLength=1  InputProcessing=Inherited  SampleTime=ts
  Math Function : Math  Operator=transpose  SaturateOnIntegerOverflow=on
  Math Function1 : Math  Operator=transpose  SaturateOnIntegerOverflow=on
  Product : Product  RndMeth=Zero
  Produto2 : Product  Inputs=**  Multiplication=Matrix(*)
  Produto3 : Product  Inputs=**  Multiplication=Matrix(*)
  Produto5 : Product  Inputs=**
  Reshape : Reshape  OutputDimensionality=Customize
  Selector : Selector  NumberOfDimensions=2  InputPortWidth=3  IndexOptions=Index vector (dialog),Select all  Indices=[2:H+1],-1  OutputSizes=1
  Wx(n+1) : Outport
  wires:
  Math Function1/1 -> Produto3/1  "Wy(n)"
  Produto3/1 -> Product/1
  Wy(n)/1 -> Math Function1/1
  Gy(n)/1 -> Reshape/1
  "[bias|X(n)]"/1 -> Math Function/1
  "[bias|Z(n)]"/1 -> Produto5/1, Gain4/1  "[bias|Z(n)]"
  Gain4/1 -> Bias2/1  "-[bias|Z(n)]"
  Bias2/1 -> Produto5/2  "1-[bias|Z(n)]"
  Produto5/1 -> Product/2  "[bias|Z(n)](1-[bias|Z(n)])"
  Product/1 -> Selector/1  "Gx(n)"
  Math Function/1 -> Produto2/2
  Selector/1 -> Produto2/1
  Gain2/1 -> Add/3  "DWx(n)"
  Integer Delay/1 -> Gain3/1
  Gain3/1 -> Add/2  "Wx(n-1)"
  Produto2/1 -> Gain2/1
  Add/1 -> Integer Delay1/1  "Wx(n+1)"
  Integer Delay1/1 -> IC/1  "Wx(n)"
  IC/1 -> Wx(n+1)/1, Add/1, Integer Delay/1
  Reshape/1 -> Produto3/2

== system Relu_OutFB_4_4_1_HW_C1/Subsystem/Backpropagation Algorithm/Output Layer ==
  "[bias|Z(n)]" : Inport
  E(n) : Inport  Port=2
  Add : Sum  Inputs=+++
  Gain2 : Gain  Gain=mu/N
  Gain3 : Gain  Gain=alpha
  IC : InitialCondition  Value=rand(m,H+1)
  IC1 : InitialCondition  Value=rand(m,H+1)
  Integer Delay : Delay  DelayLength=1  InputProcessing=Inherited  SampleTime=ts
  Integer Delay1 : Delay  DelayLength=1  InputProcessing=Inherited  SampleTime=ts
  Math Function : Math  Operator=transpose  SaturateOnIntegerOverflow=on
  Produto2 : Product  Inputs=**  Multiplication=Matrix(*)
  Wy(n+1) : Outport
  Wy(n) : Outport  Port=2
  Gy(n) : Outport  Port=3
  wires:
  "[bias|Z(n)]"/1 -> Math Function/1
  Math Function/1 -> Produto2/2
  Gain2/1 -> Add/3  "DWy(n)"
  Integer Delay/1 -> Gain3/1
  Add/1 -> Integer Delay1/1
  Gain3/1 -> Add/2  "Wy(n-1)"
  Integer Delay1/1 -> IC/1  "Wy(n+1)"
  IC/1 -> Wy(n+1)/1, Add/1, Integer Delay/1, Wy(n)/1
  Produto2/1 -> IC1/1
  IC1/1 -> Gain2/1
  E(n)/1 -> Produto2/1, Gy(n)/1  "E(n)"

== system Relu_OutFB_4_4_1_HW_C1/Subsystem/MLP - 2 Layers/Sigmoid ==
  In1 : Inport
  Bias : Bias  Bias=1
  Math Function : Math  SaturateOnIntegerOverflow=on
  Math Function1 : Math  Operator=reciprocal  SaturateOnIntegerOverflow=on
  a : Gain  Gain=-1
  Out1 : Outport
  wires:
  In1/1 -> a/1  "x"
  a/1 -> Math Function/1  "-x"
  Math Function/1 -> Bias/1  "exp(-x)"
  Bias/1 -> Math Function1/1  "1+exp(-x)"
  Math Function1/1 -> Out1/1  "1/(1+exp(-x))"

== system Relu_OutFB_4_4_1_HW_C1/EN_MLP_BK_(1,4_NL,1_L)_HW_FPGA/MLP_BK_(2,4_NL,1_L)_HW_FPGA/BK (2,4_NL,1_L)/Camada de Saída0 ==
  z_0(n) : Inport
  e(n) : Inport  Port=2
  AddSub1 : xbsIndex_r4/AddSub  mode=Addition  use_carryin=off  use_carryout=off  en=off  latency=0  precision=User Defined  arith_type="Signed  (2's comp)"  n_bits=nb  bin_pt=bp  quantization=Truncate  overflow=Wrap  dbl_ovrd=off  use_behavioral_HDL=off  hw_selection=Fabric  pipelined=off  block_type=addsub
  AddSub2 : xbsIndex_r4/AddSub  mode=Addition  use_carryin=off  use_carryout=off  en=off  latency=0  precision=User Defined  arith_type="Signed  (2's comp)"  n_bits=nb  bin_pt=bp  quantization=Truncate  overflow=Wrap  dbl_ovrd=off  use_behavioral_HDL=off  hw_selection=Fabric  pipelined=off  block_type=addsub
  CMult : xbsIndex_r4/CMult  const=mu  gui_display_data_type=Fixed-point  const_n_bits=32  const_bin_pt=32  float_type=Single  exp_bits=8  fraction_bits=24  en=off  latency=0  precision=User Defined  arith_type="Signed  (2's comp)"  n_bits=nb  bin_pt=bp  quantization="Round  (unbiased: +/- Inf)"  overflow=Wrap  dbl_ovrd=off  use_behavioral_HDL=off  mem_type=Distributed RAM  pipeline=off  block_type=cmult
  CMult1 : xbsIndex_r4/CMult  const=alpha  gui_display_data_type=Fixed-point  const_n_bits=32  const_bin_pt=32  float_type=Single  exp_bits=8  fraction_bits=24  en=off  latency=0  precision=User Defined  arith_type="Signed  (2's comp)"  n_bits=nb  bin_pt=bp  quantization="Round  (unbiased: +/- Inf)"  overflow=Wrap  dbl_ovrd=off  use_behavioral_HDL=off  mem_type=Distributed RAM  pipeline=off  block_type=cmult
  Register : xbsIndex_r4/Register  init=real(M2(1))  rst=off  en=off  dbl_ovrd=off  block_type=register
  Register1 : xbsIndex_r4/Register  init=0  rst=off  en=off  dbl_ovrd=off  block_type=register
  z_0(n)*e(n) : xbsIndex_r4/Mult  precision=User Defined  arith_type="Signed  (2's comp)"  n_bits=nb  bin_pt=bp  quantization="Round  (unbiased: +/- Inf)"  overflow=Saturate  en=off  latency=delayMuly  dbl_ovrd=off  use_behavioral_HDL=off  opt=Speed  use_embedded=on  optimum_pipeline=off  pipeline=on  use_rpm=on  placement_style=Triangular  block_type=mult
  Wy_10(n) : Outport
  wires:
  Register/1 -> Register1/1, AddSub2/1, Wy_10(n)/1  "w_ij(n)"
  CMult1/1 -> AddSub1/1  "alpha*w_ij(n-1)"
  Register1/1 -> CMult1/1  "w_ij(n-1)"
  AddSub2/1 -> Register/1  "w_ij(n+1)"
  AddSub1/1 -> AddSub2/2
  z_0(n)/1 -> z_0(n)*e(n)/1
  e(n)/1 -> z_0(n)*e(n)/2
  CMult/1 -> AddSub1/2  "dw(n) = z_0(n)*e(n)*mu"
  z_0(n)*e(n)/1 -> CMult/1

== system Relu_OutFB_4_4_1_HW_C1/EN_MLP_BK_(1,4_NL,1_L)_HW_FPGA/MLP_BK_(2,4_NL,1_L)_HW_FPGA/BK (2,4_NL,1_L)/Camada de Saída1 ==
  z_1(n) : Inport
  e(n) : Inport  Port=2
  AddSub1 : xbsIndex_r4/AddSub  mode=Addition  use_carryin=off  use_carryout=off  en=off  latency=0  precision=User Defined  arith_type="Signed  (2's comp)"  n_bits=nb  bin_pt=bp  quantization=Truncate  overflow=Wrap  dbl_ovrd=off  use_behavioral_HDL=off  hw_selection=Fabric  pipelined=off  block_type=addsub
  AddSub2 : xbsIndex_r4/AddSub  mode=Addition  use_carryin=off  use_carryout=off  en=off  latency=0  precision=User Defined  arith_type="Signed  (2's comp)"  n_bits=nb  bin_pt=bp  quantization=Truncate  overflow=Wrap  dbl_ovrd=off  use_behavioral_HDL=off  hw_selection=Fabric  pipelined=off  block_type=addsub
  CMult : xbsIndex_r4/CMult  const=mu  gui_display_data_type=Fixed-point  const_n_bits=32  const_bin_pt=32  float_type=Single  exp_bits=8  fraction_bits=24  en=off  latency=0  precision=User Defined  arith_type="Signed  (2's comp)"  n_bits=nb  bin_pt=bp  quantization="Round  (unbiased: +/- Inf)"  overflow=Wrap  dbl_ovrd=off  use_behavioral_HDL=off  mem_type=Distributed RAM  pipeline=off  block_type=cmult
  CMult1 : xbsIndex_r4/CMult  const=alpha  gui_display_data_type=Fixed-point  const_n_bits=32  const_bin_pt=32  float_type=Single  exp_bits=8  fraction_bits=24  en=off  latency=0  precision=User Defined  arith_type="Signed  (2's comp)"  n_bits=nb  bin_pt=bp  quantization="Round  (unbiased: +/- Inf)"  overflow=Wrap  dbl_ovrd=off  use_behavioral_HDL=off  mem_type=Distributed RAM  pipeline=off  block_type=cmult
  Register : xbsIndex_r4/Register  init=real(M2(2))  rst=off  en=off  dbl_ovrd=off  block_type=register
  Register1 : xbsIndex_r4/Register  init=0  rst=off  en=off  dbl_ovrd=off  block_type=register
  z_1(n)*e(n) : xbsIndex_r4/Mult  precision=User Defined  arith_type="Signed  (2's comp)"  n_bits=nb  bin_pt=bp  quantization="Round  (unbiased: +/- Inf)"  overflow=Saturate  en=off  latency=delayMuly  dbl_ovrd=off  use_behavioral_HDL=off  opt=Speed  use_embedded=on  optimum_pipeline=off  pipeline=on  use_rpm=on  placement_style=Triangular  block_type=mult
  Wy_11(n) : Outport
  Gy_11(n) : Outport  Port=2
  wires:
  Register/1 -> Register1/1, AddSub2/1, Wy_11(n)/1  "w_ij(n)"
  CMult1/1 -> AddSub1/1  "alpha*w_ij(n-1)"
  Register1/1 -> CMult1/1  "w_ij(n-1)"
  AddSub2/1 -> Register/1  "w_ij(n+1)"
  AddSub1/1 -> AddSub2/2
  z_1(n)/1 -> z_1(n)*e(n)/1
  e(n)/1 -> Gy_11(n)/1, z_1(n)*e(n)/2
  CMult/1 -> AddSub1/2  "dw(n) = z_0(n)*e(n)*mu"
  z_1(n)*e(n)/1 -> CMult/1

== system Relu_OutFB_4_4_1_HW_C1/EN_MLP_BK_(1,4_NL,1_L)_HW_FPGA/MLP_BK_(2,4_NL,1_L)_HW_FPGA/BK (2,4_NL,1_L)/Camada de Saída2 ==
  z_1(n) : Inport
  e(n) : Inport  Port=2
  AddSub1 : xbsIndex_r4/AddSub  mode=Addition  use_carryin=off  use_carryout=off  en=off  latency=0  precision=User Defined  arith_type="Signed  (2's comp)"  n_bits=nb  bin_pt=bp  quantization=Truncate  overflow=Wrap  dbl_ovrd=off  use_behavioral_HDL=off  hw_selection=Fabric  pipelined=off  block_type=addsub
  AddSub2 : xbsIndex_r4/AddSub  mode=Addition  use_carryin=off  use_carryout=off  en=off  latency=0  precision=User Defined  arith_type="Signed  (2's comp)"  n_bits=nb  bin_pt=bp  quantization=Truncate  overflow=Wrap  dbl_ovrd=off  use_behavioral_HDL=off  hw_selection=Fabric  pipelined=off  block_type=addsub
  CMult : xbsIndex_r4/CMult  const=mu  gui_display_data_type=Fixed-point  const_n_bits=32  const_bin_pt=32  float_type=Single  exp_bits=8  fraction_bits=24  en=off  latency=0  precision=User Defined  arith_type="Signed  (2's comp)"  n_bits=nb  bin_pt=bp  quantization="Round  (unbiased: +/- Inf)"  overflow=Wrap  dbl_ovrd=off  use_behavioral_HDL=off  mem_type=Distributed RAM  pipeline=off  block_type=cmult
  CMult1 : xbsIndex_r4/CMult  const=alpha  gui_display_data_type=Fixed-point  const_n_bits=32  const_bin_pt=32  float_type=Single  exp_bits=8  fraction_bits=24  en=off  latency=0  precision=User Defined  arith_type="Signed  (2's comp)"  n_bits=nb  bin_pt=bp  quantization="Round  (unbiased: +/- Inf)"  overflow=Wrap  dbl_ovrd=off  use_behavioral_HDL=off  mem_type=Distributed RAM  pipeline=off  block_type=cmult
  Register : xbsIndex_r4/Register  init=real(M2(4))  rst=off  en=off  dbl_ovrd=off  block_type=register
  Register1 : xbsIndex_r4/Register  init=0  rst=off  en=off  dbl_ovrd=off  block_type=register
  z_1(n)*e(n) : xbsIndex_r4/Mult  precision=User Defined  arith_type="Signed  (2's comp)"  n_bits=nb  bin_pt=bp  quantization="Round  (unbiased: +/- Inf)"  overflow=Saturate  en=off  latency=delayMuly  dbl_ovrd=off  use_behavioral_HDL=off  opt=Speed  use_embedded=on  optimum_pipeline=off  pipeline=on  use_rpm=on  placement_style=Triangular  block_type=mult
  Wy_11(n) : Outport
  Gy_11(n) : Outport  Port=2
  wires:
  Register/1 -> Register1/1, AddSub2/1, Wy_11(n)/1  "w_ij(n)"
  CMult1/1 -> AddSub1/1  "alpha*w_ij(n-1)"
  Register1/1 -> CMult1/1  "w_ij(n-1)"
  AddSub2/1 -> Register/1  "w_ij(n+1)"
  AddSub1/1 -> AddSub2/2
  z_1(n)/1 -> z_1(n)*e(n)/1
  e(n)/1 -> Gy_11(n)/1, z_1(n)*e(n)/2
  CMult/1 -> AddSub1/2  "dw(n) = z_0(n)*e(n)*mu"
  z_1(n)*e(n)/1 -> CMult/1

== system Relu_OutFB_4_4_1_HW_C1/EN_MLP_BK_(1,4_NL,1_L)_HW_FPGA/MLP_BK_(2,4_NL,1_L)_HW_FPGA/BK (2,4_NL,1_L)/Camada de Saída3 ==
  z_1(n) : Inport
  e(n) : Inport  Port=2
  AddSub1 : xbsIndex_r4/AddSub  mode=Addition  use_carryin=off  use_carryout=off  en=off  latency=0  precision=User Defined  arith_type="Signed  (2's comp)"  n_bits=nb  bin_pt=bp  quantization=Truncate  overflow=Wrap  dbl_ovrd=off  use_behavioral_HDL=off  hw_selection=Fabric  pipelined=off  block_type=addsub
  AddSub2 : xbsIndex_r4/AddSub  mode=Addition  use_carryin=off  use_carryout=off  en=off  latency=0  precision=User Defined  arith_type="Signed  (2's comp)"  n_bits=nb  bin_pt=bp  quantization=Truncate  overflow=Wrap  dbl_ovrd=off  use_behavioral_HDL=off  hw_selection=Fabric  pipelined=off  block_type=addsub
  CMult : xbsIndex_r4/CMult  const=mu  gui_display_data_type=Fixed-point  const_n_bits=32  const_bin_pt=32  float_type=Single  exp_bits=8  fraction_bits=24  en=off  latency=0  precision=User Defined  arith_type="Signed  (2's comp)"  n_bits=nb  bin_pt=bp  quantization="Round  (unbiased: +/- Inf)"  overflow=Wrap  dbl_ovrd=off  use_behavioral_HDL=off  mem_type=Distributed RAM  pipeline=off  block_type=cmult
  CMult1 : xbsIndex_r4/CMult  const=alpha  gui_display_data_type=Fixed-point  const_n_bits=32  const_bin_pt=32  float_type=Single  exp_bits=8  fraction_bits=24  en=off  latency=0  precision=User Defined  arith_type="Signed  (2's comp)"  n_bits=nb  bin_pt=bp  quantization="Round  (unbiased: +/- Inf)"  overflow=Wrap  dbl_ovrd=off  use_behavioral_HDL=off  mem_type=Distributed RAM  pipeline=off  block_type=cmult
  Register : xbsIndex_r4/Register  init=real(M2(3))  rst=off  en=off  dbl_ovrd=off  block_type=register
  Register1 : xbsIndex_r4/Register  init=0  rst=off  en=off  dbl_ovrd=off  block_type=register
  z_1(n)*e(n) : xbsIndex_r4/Mult  precision=User Defined  arith_type="Signed  (2's comp)"  n_bits=nb  bin_pt=bp  quantization="Round  (unbiased: +/- Inf)"  overflow=Saturate  en=off  latency=delayMuly  dbl_ovrd=off  use_behavioral_HDL=off  opt=Speed  use_embedded=on  optimum_pipeline=off  pipeline=on  use_rpm=on  placement_style=Triangular  block_type=mult
  Wy_11(n) : Outport
  Gy_11(n) : Outport  Port=2
  wires:
  z_1(n)*e(n)/1 -> CMult/1
  CMult/1 -> AddSub1/2  "dw(n) = z_0(n)*e(n)*mu"
  e(n)/1 -> z_1(n)*e(n)/2, Gy_11(n)/1
  z_1(n)/1 -> z_1(n)*e(n)/1
  AddSub1/1 -> AddSub2/2
  AddSub2/1 -> Register/1  "w_ij(n+1)"
  Register1/1 -> CMult1/1  "w_ij(n-1)"
  CMult1/1 -> AddSub1/1  "alpha*w_ij(n-1)"
  Register/1 -> Wy_11(n)/1, AddSub2/1, Register1/1  "w_ij(n)"

== system Relu_OutFB_4_4_1_HW_C1/EN_MLP_BK_(1,4_NL,1_L)_HW_FPGA/MLP_BK_(2,4_NL,1_L)_HW_FPGA/BK (2,4_NL,1_L)/Camada de Saída4 ==
  z_1(n) : Inport
  e(n) : Inport  Port=2
  AddSub1 : xbsIndex_r4/AddSub  mode=Addition  use_carryin=off  use_carryout=off  en=off  latency=0  precision=User Defined  arith_type="Signed  (2's comp)"  n_bits=nb  bin_pt=bp  quantization=Truncate  overflow=Wrap  dbl_ovrd=off  use_behavioral_HDL=off  hw_selection=Fabric  pipelined=off  block_type=addsub
  AddSub2 : xbsIndex_r4/AddSub  mode=Addition  use_carryin=off  use_carryout=off  en=off  latency=0  precision=User Defined  arith_type="Signed  (2's comp)"  n_bits=nb  bin_pt=bp  quantization=Truncate  overflow=Wrap  dbl_ovrd=off  use_behavioral_HDL=off  hw_selection=Fabric  pipelined=off  block_type=addsub
  CMult : xbsIndex_r4/CMult  const=mu  gui_display_data_type=Fixed-point  const_n_bits=32  const_bin_pt=32  float_type=Single  exp_bits=8  fraction_bits=24  en=off  latency=0  precision=User Defined  arith_type="Signed  (2's comp)"  n_bits=nb  bin_pt=bp  quantization="Round  (unbiased: +/- Inf)"  overflow=Wrap  dbl_ovrd=off  use_behavioral_HDL=off  mem_type=Distributed RAM  pipeline=off  block_type=cmult
  CMult1 : xbsIndex_r4/CMult  const=alpha  gui_display_data_type=Fixed-point  const_n_bits=32  const_bin_pt=32  float_type=Single  exp_bits=8  fraction_bits=24  en=off  latency=0  precision=User Defined  arith_type="Signed  (2's comp)"  n_bits=nb  bin_pt=bp  quantization="Round  (unbiased: +/- Inf)"  overflow=Wrap  dbl_ovrd=off  use_behavioral_HDL=off  mem_type=Distributed RAM  pipeline=off  block_type=cmult
  Register : xbsIndex_r4/Register  init=real(M2(5))  rst=off  en=off  dbl_ovrd=off  block_type=register
  Register1 : xbsIndex_r4/Register  init=0  rst=off  en=off  dbl_ovrd=off  block_type=register
  z_1(n)*e(n) : xbsIndex_r4/Mult  precision=User Defined  arith_type="Signed  (2's comp)"  n_bits=nb  bin_pt=bp  quantization="Round  (unbiased: +/- Inf)"  overflow=Saturate  en=off  latency=delayMuly  dbl_ovrd=off  use_behavioral_HDL=off  opt=Speed  use_embedded=on  optimum_pipeline=off  pipeline=on  use_rpm=on  placement_style=Triangular  block_type=mult
  Wy_11(n) : Outport
  Gy_11(n) : Outport  Port=2
  wires:
  z_1(n)*e(n)/1 -> CMult/1
  CMult/1 -> AddSub1/2  "dw(n) = z_0(n)*e(n)*mu"
  e(n)/1 -> z_1(n)*e(n)/2, Gy_11(n)/1
  z_1(n)/1 -> z_1(n)*e(n)/1
  AddSub1/1 -> AddSub2/2
  AddSub2/1 -> Register/1  "w_ij(n+1)"
  Register1/1 -> CMult1/1  "w_ij(n-1)"
  CMult1/1 -> AddSub1/1  "alpha*w_ij(n-1)"
  Register/1 -> Wy_11(n)/1, AddSub2/1, Register1/1  "w_ij(n)"

== system Relu_OutFB_4_4_1_HW_C1/EN_MLP_BK_(1,4_NL,1_L)_HW_FPGA/MLP_BK_(2,4_NL,1_L)_HW_FPGA/BK (2,4_NL,1_L)/Subsystem1 ==
  z_1(n) : Inport
  Wy_11(n) : Inport  Port=2
  Gy_11(n) : Inport  Port=3
  Constant : xbsIndex_r4/Constant  const=0  gui_display_data_type=Fixed-point  arith_type=Signed (2's comp)  n_bits=nb  bin_pt=bp  preci_type=Single  exp_width=8  frac_width=24  explicit_period=off  period=1  equ=P=C  opselect=C  inp2=PCIN>>17  opr=+  inp1=P  carry=CIN  dbl_ovrd=off  block_type=constant
  Reinterpret : xbsIndex_r4/Reinterpret  force_arith_type=on  arith_type="Signed  (2's comp)"  force_bin_pt=on  bin_pt=0  block_type=reinterpret
  Relational : xbsIndex_r4/Relational  mode=a<=b  en=off  latency=0  dbl_ovrd=off  block_type=relational
  w_ij(n)*Gy(n) : xbsIndex_r4/Mult  precision=User Defined  arith_type="Signed  (2's comp)"  n_bits=nb  bin_pt=bp  quantization="Round  (unbiased: +/- Inf)"  overflow=Saturate  en=off  latency=delayMuly  dbl_ovrd=off  use_behavioral_HDL=off  opt=Speed  use_embedded=on  optimum_pipeline=off  pipeline=on  use_rpm=on  placement_style=Triangular  block_type=mult
  w_ij(n)*Gy(n)1 : xbsIndex_r4/Mult  precision=User Defined  arith_type="Signed  (2's comp)"  n_bits=nb  bin_pt=bp  quantization="Round  (unbiased: +/- Inf)"  overflow=Saturate  en=off  latency=delayMuly  dbl_ovrd=off  use_behavioral_HDL=off  opt=Speed  use_embedded=on  optimum_pipeline=off  pipeline=on  use_rpm=on  placement_style=Triangular  block_type=mult
  Gx_1(n) : Outport
  wires:
  w_ij(n)*Gy(n)1/1 -> Gx_1(n)/1
  Relational/1 -> Reinterpret/1
  Gy_11(n)/1 -> w_ij(n)*Gy(n)/2
  w_ij(n)*Gy(n)/1 -> w_ij(n)*Gy(n)1/2
  Wy_11(n)/1 -> w_ij(n)*Gy(n)/1
  Constant/1 -> Relational/2
  z_1(n)/1 -> Relational/1
  Reinterpret/1 -> w_ij(n)*Gy(n)1/1

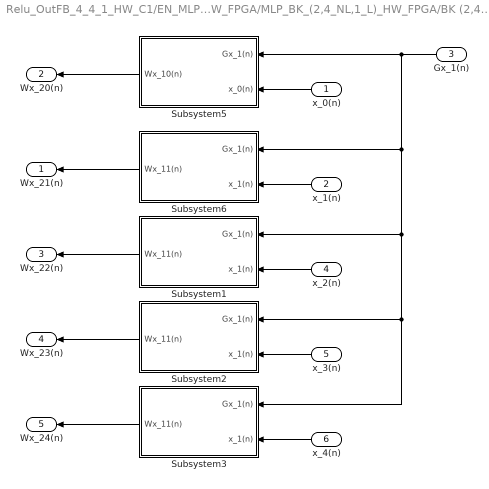
== system Relu_OutFB_4_4_1_HW_C1/EN_MLP_BK_(1,4_NL,1_L)_HW_FPGA/MLP_BK_(2,4_NL,1_L)_HW_FPGA/BK (2,4_NL,1_L)/Subsystem2 ==
  x_0(n) : Inport
  x_1(n) : Inport  Port=2
  Gx_1(n) : Inport  Port=3
  x_2(n) : Inport  Port=4
  x_3(n) : Inport  Port=5
  x_4(n) : Inport  Port=6
  Subsystem1 : Subsystem
  Subsystem2 : Subsystem
  Subsystem3 : Subsystem
  Subsystem5 : Subsystem
  Subsystem6 : Subsystem
  Wx_21(n) : Outport
  Wx_20(n) : Outport  Port=2
  Wx_22(n) : Outport  Port=3
  Wx_23(n) : Outport  Port=4
  Wx_24(n) : Outport  Port=5
  wires:
  Subsystem3/1(Wx_11(n)) -> Wx_24(n)/1
  x_4(n)/1 -> Subsystem3/2(x_1(n))
  Gx_1(n)/1 -> Subsystem6/1(Gx_1(n)), Subsystem1/1(Gx_1(n)), Subsystem2/1(Gx_1(n)), Subsystem3/1(Gx_1(n)), Subsystem5/1(Gx_1(n))
  Subsystem1/1(Wx_11(n)) -> Wx_22(n)/1
  Subsystem2/1(Wx_11(n)) -> Wx_23(n)/1
  x_2(n)/1 -> Subsystem1/2(x_1(n))
  x_3(n)/1 -> Subsystem2/2(x_1(n))
  x_1(n)/1 -> Subsystem6/2(x_1(n))
  Subsystem6/1(Wx_11(n)) -> Wx_21(n)/1
  x_0(n)/1 -> Subsystem5/2(x_0(n))
  Subsystem5/1(Wx_10(n)) -> Wx_20(n)/1

== system Relu_OutFB_4_4_1_HW_C1/EN_MLP_BK_(1,4_NL,1_L)_HW_FPGA/MLP_BK_(2,4_NL,1_L)_HW_FPGA/BK (2,4_NL,1_L)/Subsystem3 ==
  z_1(n) : Inport
  Wy_11(n) : Inport  Port=2
  Gy_11(n) : Inport  Port=3
  Constant : xbsIndex_r4/Constant  const=0  gui_display_data_type=Fixed-point  arith_type=Signed (2's comp)  n_bits=nb  bin_pt=bp  preci_type=Single  exp_width=8  frac_width=24  explicit_period=off  period=1  equ=P=C  opselect=C  inp2=PCIN>>17  opr=+  inp1=P  carry=CIN  dbl_ovrd=off  block_type=constant
  Reinterpret : xbsIndex_r4/Reinterpret  force_arith_type=on  arith_type="Signed  (2's comp)"  force_bin_pt=on  bin_pt=0  block_type=reinterpret
  Relational : xbsIndex_r4/Relational  mode=a<=b  en=off  latency=0  dbl_ovrd=off  block_type=relational
  w_ij(n)*Gy(n) : xbsIndex_r4/Mult  precision=User Defined  arith_type="Signed  (2's comp)"  n_bits=nb  bin_pt=bp  quantization="Round  (unbiased: +/- Inf)"  overflow=Saturate  en=off  latency=delayMuly  dbl_ovrd=off  use_behavioral_HDL=off  opt=Speed  use_embedded=on  optimum_pipeline=off  pipeline=on  use_rpm=on  placement_style=Triangular  block_type=mult
  w_ij(n)*Gy(n)1 : xbsIndex_r4/Mult  precision=User Defined  arith_type="Signed  (2's comp)"  n_bits=nb  bin_pt=bp  quantization="Round  (unbiased: +/- Inf)"  overflow=Saturate  en=off  latency=delayMuly  dbl_ovrd=off  use_behavioral_HDL=off  opt=Speed  use_embedded=on  optimum_pipeline=off  pipeline=on  use_rpm=on  placement_style=Triangular  block_type=mult
  Gx_1(n) : Outport
  wires:
  w_ij(n)*Gy(n)1/1 -> Gx_1(n)/1
  Relational/1 -> Reinterpret/1
  Gy_11(n)/1 -> w_ij(n)*Gy(n)/2
  w_ij(n)*Gy(n)/1 -> w_ij(n)*Gy(n)1/2
  Wy_11(n)/1 -> w_ij(n)*Gy(n)/1
  Constant/1 -> Relational/2
  z_1(n)/1 -> Relational/1
  Reinterpret/1 -> w_ij(n)*Gy(n)1/1

== system Relu_OutFB_4_4_1_HW_C1/EN_MLP_BK_(1,4_NL,1_L)_HW_FPGA/MLP_BK_(2,4_NL,1_L)_HW_FPGA/BK (2,4_NL,1_L)/Subsystem4 ==
  z_1(n) : Inport
  Wy_11(n) : Inport  Port=2
  Gy_11(n) : Inport  Port=3
  Constant : xbsIndex_r4/Constant  const=0  gui_display_data_type=Fixed-point  arith_type=Signed (2's comp)  n_bits=nb  bin_pt=bp  preci_type=Single  exp_width=8  frac_width=24  explicit_period=off  period=1  equ=P=C  opselect=C  inp2=PCIN>>17  opr=+  inp1=P  carry=CIN  dbl_ovrd=off  block_type=constant
  Reinterpret : xbsIndex_r4/Reinterpret  force_arith_type=on  arith_type="Signed  (2's comp)"  force_bin_pt=on  bin_pt=0  block_type=reinterpret
  Relational : xbsIndex_r4/Relational  mode=a<=b  en=off  latency=0  dbl_ovrd=off  block_type=relational
  w_ij(n)*Gy(n) : xbsIndex_r4/Mult  precision=User Defined  arith_type="Signed  (2's comp)"  n_bits=nb  bin_pt=bp  quantization="Round  (unbiased: +/- Inf)"  overflow=Saturate  en=off  latency=delayMuly  dbl_ovrd=off  use_behavioral_HDL=off  opt=Speed  use_embedded=on  optimum_pipeline=off  pipeline=on  use_rpm=on  placement_style=Triangular  block_type=mult
  w_ij(n)*Gy(n)1 : xbsIndex_r4/Mult  precision=User Defined  arith_type="Signed  (2's comp)"  n_bits=nb  bin_pt=bp  quantization="Round  (unbiased: +/- Inf)"  overflow=Saturate  en=off  latency=delayMuly  dbl_ovrd=off  use_behavioral_HDL=off  opt=Speed  use_embedded=on  optimum_pipeline=off  pipeline=on  use_rpm=on  placement_style=Triangular  block_type=mult
  Gx_1(n) : Outport
  wires:
  w_ij(n)*Gy(n)1/1 -> Gx_1(n)/1
  Relational/1 -> Reinterpret/1
  Gy_11(n)/1 -> w_ij(n)*Gy(n)/2
  w_ij(n)*Gy(n)/1 -> w_ij(n)*Gy(n)1/2
  Wy_11(n)/1 -> w_ij(n)*Gy(n)/1
  Constant/1 -> Relational/2
  z_1(n)/1 -> Relational/1
  Reinterpret/1 -> w_ij(n)*Gy(n)1/1

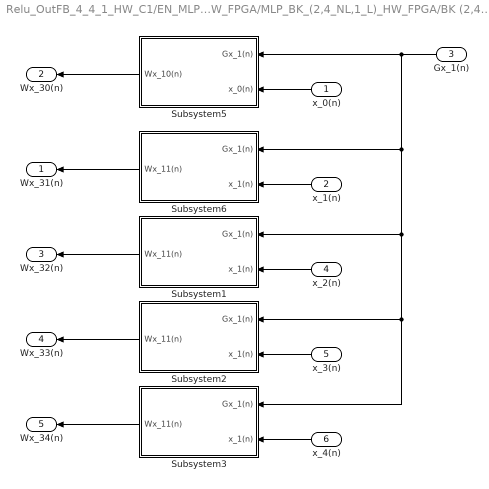
== system Relu_OutFB_4_4_1_HW_C1/EN_MLP_BK_(1,4_NL,1_L)_HW_FPGA/MLP_BK_(2,4_NL,1_L)_HW_FPGA/BK (2,4_NL,1_L)/Subsystem5 ==
  x_0(n) : Inport
  x_1(n) : Inport  Port=2
  Gx_1(n) : Inport  Port=3
  x_2(n) : Inport  Port=4
  x_3(n) : Inport  Port=5
  x_4(n) : Inport  Port=6
  Subsystem1 : Subsystem
  Subsystem2 : Subsystem
  Subsystem3 : Subsystem
  Subsystem5 : Subsystem
  Subsystem6 : Subsystem
  Wx_31(n) : Outport
  Wx_30(n) : Outport  Port=2
  Wx_32(n) : Outport  Port=3
  Wx_33(n) : Outport  Port=4
  Wx_34(n) : Outport  Port=5
  wires:
  Subsystem5/1(Wx_10(n)) -> Wx_30(n)/1
  x_0(n)/1 -> Subsystem5/2(x_0(n))
  Subsystem6/1(Wx_11(n)) -> Wx_31(n)/1
  x_1(n)/1 -> Subsystem6/2(x_1(n))
  x_3(n)/1 -> Subsystem2/2(x_1(n))
  x_2(n)/1 -> Subsystem1/2(x_1(n))
  Subsystem2/1(Wx_11(n)) -> Wx_33(n)/1
  Subsystem1/1(Wx_11(n)) -> Wx_32(n)/1
  Gx_1(n)/1 -> Subsystem5/1(Gx_1(n)), Subsystem3/1(Gx_1(n)), Subsystem2/1(Gx_1(n)), Subsystem1/1(Gx_1(n)), Subsystem6/1(Gx_1(n))
  x_4(n)/1 -> Subsystem3/2(x_1(n))
  Subsystem3/1(Wx_11(n)) -> Wx_34(n)/1
